simulink model "Enable_Trigger_subsystem"  (R2018b)
settings: Solver=FixedStepDiscrete  StartTime=0.0  StopTime=14  RelTol=1e-3
libraries: simulink x1
settings Model: Creator=marwan  LastModifiedBy=marwan

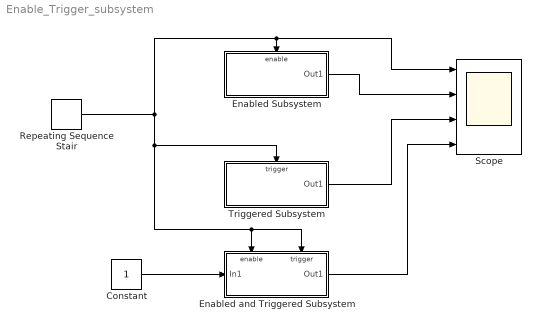
== system Enable_Trigger_subsystem ==
  Constant : Constant
  Enabled Subsystem : Subsystem  TreatAsAtomicUnit=on
  Enabled and Triggered Subsystem : Subsystem  TreatAsAtomicUnit=on
  Repeating Sequence Stair : simulink/Sources/Repeating Sequence Stair  OutValues=[0 0 0 1 0 1 1 1 0 0 0 1 1 0]  tsamp=-1  OutMin=[]  OutMax=[]  OutDataTypeStr=double  OutputDataTypeScalingMode=double  OutDataType=fixdt(0,8)  ConRadixGroup=Best Precision: Vector-wise  OutScaling=2^-12
  Scope : Scope  NumInputPorts=4
  Triggered Subsystem : Subsystem  TreatAsAtomicUnit=on
  wires:
  Repeating Sequence Stair/1 -> Enabled and Triggered Subsystem/Enable, Enabled and Triggered Subsystem/Trigger, Triggered Subsystem/Trigger, Scope/1, Enabled Subsystem/Enable
  Enabled Subsystem/1(Out1) -> Scope/2
  Triggered Subsystem/1(Out1) -> Scope/3
  Constant/1 -> Enabled and Triggered Subsystem/1(In1)
  Enabled and Triggered Subsystem/1(Out1) -> Scope/4

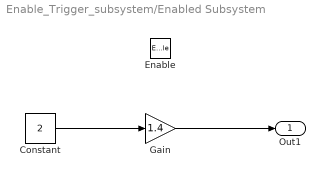
== system Enable_Trigger_subsystem/Enabled Subsystem ==
  Enable : EnablePort  StatesWhenEnabling=reset
  Constant : Constant  Value=2
  Gain : Gain  Gain=1.4
  Out1 : Outport  OutputWhenDisabled=reset  InitialOutput=[0]
  wires:
  Constant/1 -> Gain/1
  Gain/1 -> Out1/1

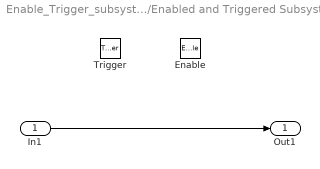
== system Enable_Trigger_subsystem/Enabled and Triggered Subsystem ==
  In1 : Inport
  Enable : EnablePort
  Trigger : TriggerPort  VariantControl=Variant
  Out1 : Outport
  wires:
  In1/1 -> Out1/1

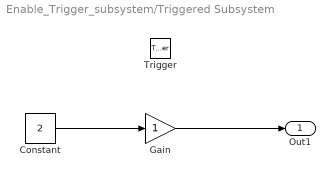
== system Enable_Trigger_subsystem/Triggered Subsystem ==
  Trigger : TriggerPort  TriggerType=falling  VariantControl=Variant  InitialTriggerSignalState=zero
  Constant : Constant  Value=2
  Gain : Gain
  Out1 : Outport  InitialOutput=[0]
  wires:
  Gain/1 -> Out1/1
  Constant/1 -> Gain/1
